simulink model "Maglev"  (Simulink 7.7)
settings: Solver=ode45  StartTime=0.0  StopTime=10.0  RelTol=1e-3
values from neighbouring files (symbols this model uses):
  C = 1    [MagLevInit.m]
  R1 = 46.2e3    (= 46200)    [MagLevInit.m]
  R2 = 999    [MagLevInit.m]
  rbeam = (1.5048/1000)    (= 0.0015048)    [MagLevInit.m]
  rblock = (6.35/1000)    (= 0.00635)    [MagLevInit.m]
  Rs = 0.5    [MagLevInit.m]
undefined symbols (not defined in the file or in its folder): g, m
settings Model: Creator=gshiva  LastModifiedBy=gshiva

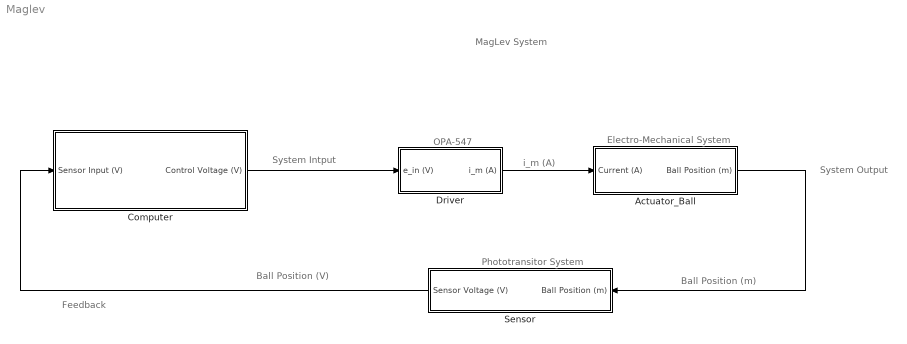
== system Maglev ==
  note: i_m (A)
  note: Ball Position (m)
  note: Ball Position (V)
  note: OPA-547
  note: Electro-Mechanical System
  note: Phototransitor System
  note: System Output
  note: MagLev System
  note: System Intput
  note: Feedback
  Actuator_Ball : Subsystem
  Computer : Subsystem
  Driver : Subsystem
  Sensor : Subsystem
  wires:
  Computer/1(Control Voltage (V)) -> Driver/1(e_in (V))
  Driver/1(i_m (A)) -> Actuator_Ball/1(Current (A))
  Actuator_Ball/1(Ball Position (m)) -> Sensor/1(Ball Position (m))
  Sensor/1(Sensor Voltage (V)) -> Computer/1(Sensor Input (V))

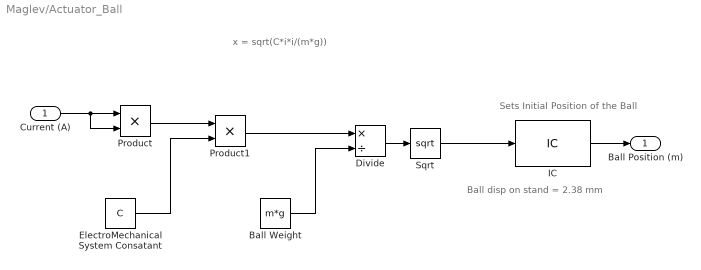
== system Maglev/Actuator_Ball ==
  note: x = sqrt(C*i*i/(m*g))
  note: Sets Initial Position of the Ball
  note: Ball disp on stand = 2.38 mm
  Current (A) : Inport
  Ball Weight : Constant  Value=m*g
  Divide : Product  Inputs=*/
  ElectroMechanical System Consatant : Constant  Value=C
  IC : InitialCondition  Value=(2.38/1000)
  Product : Product  RndMeth=Zero
  Product1 : Product  RndMeth=Zero
  Sqrt : Sqrt  SaturateOnIntegerOverflow=on
  Ball Position (m) : Outport
  wires:
  Current (A)/1 -> Product/1, Product/2
  Product/1 -> Product1/1
  ElectroMechanical System Consatant/1 -> Product1/2
  Product1/1 -> Divide/1
  Ball Weight/1 -> Divide/2
  Divide/1 -> Sqrt/1
  Sqrt/1 -> IC/1
  IC/1 -> Ball Position (m)/1

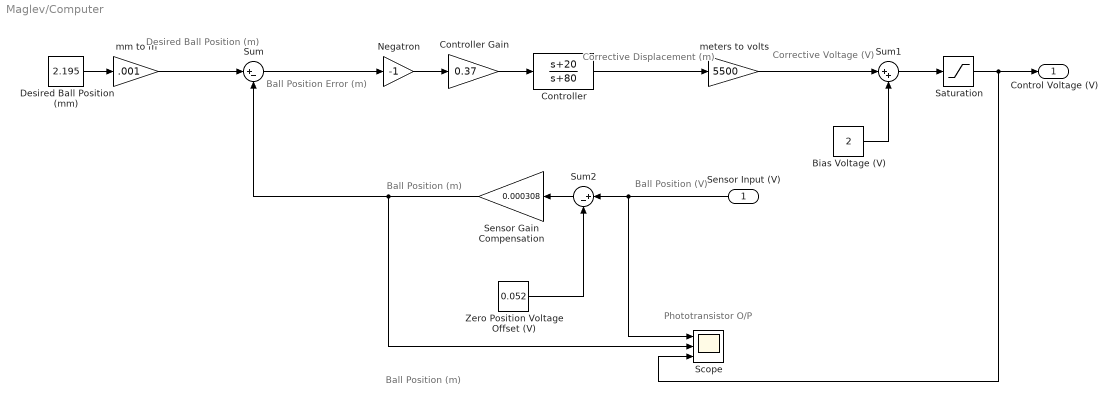
== system Maglev/Computer ==
  note: Ball Position (m)
  note: Ball Position
      | Error (m)
  note: Ball
      | Position (V)
  note: Corrective
      | Voltage (V)
  note: Corrective
      | Displacement (m)
  note: Desired Ball
      | Position (m)
  note: Phototransistor O/P
  note: Ball Position (m)
  Sensor Input (V) : Inport
  Bias Voltage (V) : Constant  Value=2
  Controller : TransferFcn  Numerator=[1 20]  Denominator=[1 80]
  Controller Gain : Gain  Gain=0.37
  Desired Ball Position (mm) : Constant  Value=2.195
  Negatron : Gain  Gain=-1
  Saturation : Saturate  UpperLimit=5  LowerLimit=0
  Scope : Scope  NumInputPorts=3
      settings: TimeRange=10  YMin=-5~-5~-5  YMax=5~5~5
  Sensor Gain Compensation : Gain  Gain=0.000308
  Sum : Sum  Inputs=|+-
  Sum1 : Sum  Inputs=|++  InputSameDT=on
  Sum2 : Sum  Inputs=|+-
  Zero Position Voltage Offset (V) : Constant  Value=0.052
  meters to volts : Gain  Gain=5500
  mm to m : Gain  Gain=.001
  Control Voltage (V) : Outport
  wires:
  Sum/1 -> Negatron/1
  Bias Voltage (V)/1 -> Sum1/2
  Sum1/1 -> Saturation/1
  Sensor Input (V)/1 -> Sum2/1, Scope/1
  Sum2/1 -> Sensor Gain Compensation/1
  Zero Position Voltage Offset (V)/1 -> Sum2/2
  Sensor Gain Compensation/1 -> Sum/2, Scope/2
  Controller/1 -> meters to volts/1
  meters to volts/1 -> Sum1/1
  Desired Ball Position (mm)/1 -> mm to m/1
  mm to m/1 -> Sum/1
  Saturation/1 -> Control Voltage (V)/1, Scope/3
  Controller Gain/1 -> Controller/1
  Negatron/1 -> Controller Gain/1

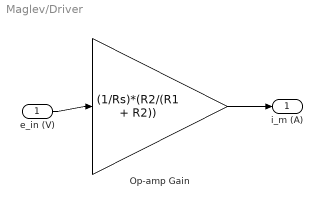
== system Maglev/Driver ==
  e_in (V) : Inport
  Op-amp Gain : Gain  Gain=(1/Rs)*(R2/(R1 + R2))
  i_m (A) : Outport
  wires:
  e_in (V)/1 -> Op-amp Gain/1
  Op-amp Gain/1 -> i_m (A)/1

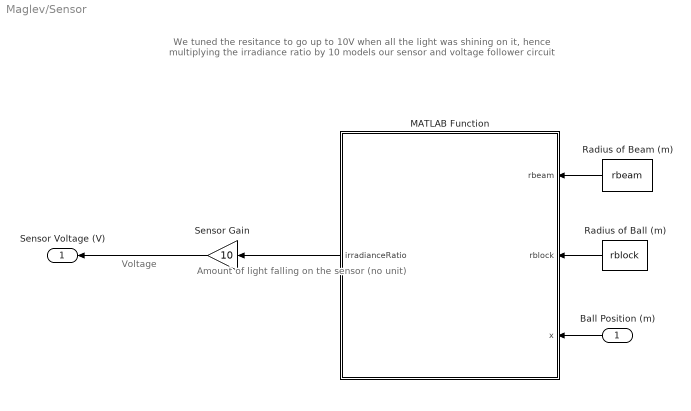
== system Maglev/Sensor ==
  note: Amount of
      | light falling
      | on the
      | sensor
      | (no unit)
  note: Voltage
  note: We tuned the resitance to go up to 10V when all the light was shining on it, hence
      |  multiplying the irradiance ratio by 10 models our sensor and voltage follower circuit
  Ball Position (m) : Inport
  MATLAB Function : Stateflow chart  TreatAsAtomicUnit=on
  Radius of Ball (m) : Constant  Value=rblock
  Radius of Beam (m) : Constant  Value=rbeam
  Sensor Gain : Gain  Gain=10
  Sensor Voltage (V) : Outport
  wires:
  Ball Position (m)/1 -> MATLAB Function/3(x)
  Radius of Beam (m)/1 -> MATLAB Function/1(rbeam)
  Radius of Ball (m)/1 -> MATLAB Function/2(rblock)
  MATLAB Function/1(irradianceRatio) -> Sensor Gain/1
  Sensor Gain/1 -> Sensor Voltage (V)/1

== matlab function Sensor/MATLAB Function ==
  data: rbeam input double; irradianceRatio output double; rblock input double; x input double
function irradianceRatio  = irradianceEstimator(rbeam, rblock, x)
% computes the fraction of irradiance as a function of the radii of the two
% intersecting circles and the distance between their centers, d
% This can be used to model the irradiance of our phototransistor if we
% make several assumptions:
% - ignore diffraction
% - assume parallel light rays from LED to photo transistor so that we can
% model the * note we should use the minimum radius of the LED and the
% phototransistor - since - the parallel ray assumption means that distance
% from the ball to the LED doesn't matter

% let r1 be the beam radius and r2 be the blocking radius

% details at http://mathworld.wolfram.com/Circle-CircleIntersection.html

% estimated rblock = 6.35 mm
% estimated rbeam as = 2.3650 mm radius of the phototransistor

% regressed rbeam = 1.5048

assert((rbeam >= 0) && (rblock >= 0), 'The radii should be non-negative');

r1 = rbeam;
r2 = rblock;

d = x - (2.23/1000);

if ((r1 > r2) && ((r2 + abs(d)) < r1))
    % handle the block is completely in the beam and the beam is bigger
    A1 = pi * r1 * r1;
    A2 = pi * r2 * r2;
    
    irradianceRatio = (A1 - A2) / A1;
    
elseif ((r2 >= r1) && ((r1 + abs(d)) <= r2))
    % handle case where block is larger or same size than beam and completely in the way
    irradianceRatio = 0;
        
elseif (abs(d) < (r1 + r2))
    % handle case where two circles intersect each other
    x = (d * d + r1 * r1 - r2 * r2) / (2 * d);
    
    d1 = x;
    d2 = (d * d - r1 * r1 + r2 * r2) / (2 * d);
    
    A = cSarea(r1, d1) + cSarea(r2, d2);
    
    Amax = pi * r1 * r1;
    
    irradianceRatio = (Amax - A) / Amax;

else 
    % handle case with no overlap
    irradianceRatio = 1;
end

end

function [area] = cSarea(r, h) 
% computes the area of the circular segment where the upper boundary is a
% circular arc and the lower boundary is a cord of the circle with radius r
% h is the perpendicular distance from the center to the cord

area = r * r * acos(h / r) - h * sqrt(r * r - h * h);

end
